simulink model "UDP_11"  (R2013b)
settings: Solver=ode45  StartTime=0.0  StopTime=1000  MaxStep=0.01  MinStep=0.01  RelTol=1e-3
libraries: dspnetwork x1, xpclib x1
settings Model: Creator=lankuohsing  LastModifiedBy=lankuohsing
settings SolverCC: InitialStep=0.01

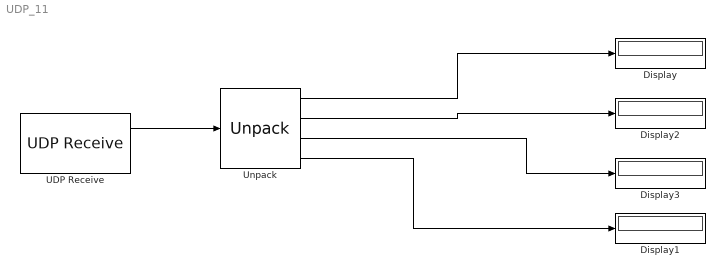
== system UDP_11 ==
  Display{,1..3} (4 alike) : Display
      settings: Decimation=100
  UDP Receive : dspnetwork/UDP Receive  localURL='0.0.0.0'  localPort=9090  remoteURL='0.0.0.0'  remotePort=-1  recvBufferSize=819200  dims=255  signalDatatype=double  isVarSize=off  showBlockingTime=on  blockingTime=inf  sampletime=0.01  blockPlatform=HOST
  Unpack : xpclib/UDP/Unpack  dimensions={[1],[1],[1],[1]}  datatypes={'double','double','double','double'}  byteAlign=1
  wires:
  Unpack/1 -> Display/1
  Unpack/2 -> Display2/1
  Unpack/3 -> Display3/1
  Unpack/4 -> Display1/1
  ? -> ?
  UDP Receive/1 -> Unpack/1
